simulink library "RLSUpdate_ul"  (R2018a)
settings: Solver=VariableStepAuto  StartTime=0.0  StopTime=10.0  RelTol=1e-3
undefined symbols (not defined in the file or in its folder): p
settings Model: Creator=mitch  LastModifiedBy=mitch

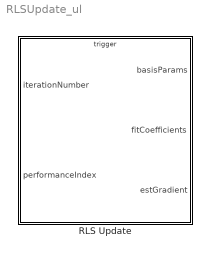
== system RLSUpdate_ul ==
  RLS Update : Subsystem  TreatAsAtomicUnit=on  mask{settlingBasisParameter=0, initializationBasisParameters=p.initializationBasisParameters*pi/180, numSettlingLaps=p.numSettlingLaps, forgettingFactor=p.forgettingFactor, normalizationFactors=p.basisParameterNormalizationFactors'*pi/180, trustRegionDimensions=p.trustRegionDimensions'*pi/180, learningGain=p.KLearningGradient, noiseAmplitude=0}
      mask prompts: settlingBasisParameter "Settling Basis Parameters"; initializationBasisParameters "Initialization Basis Parameters"; numSettlingLaps "Number of Settling Laps"; forgettingFactor "Forgetting Factor"; normalizationFactors "Basis Parameter Normalization Factors"; trustRegionDimensions "Trust Region Dimensions"; learningGain "Learning Gain"; noiseAmplitude "Noise Amplitudes"
      mask help:
      | Block implementing my RLS update
      | All vectors must be columns
      | See help for detailed description of inputs
      mask Help:
      | RLS update of the basis parameters using a quadratic regressor vector and gradient based update with a trust region.
      | let N be the number of basis parameters and M be the number of points in basis parameter design space used to initialize the algorithm
      | 
      | INPUTS :
      | Initialization basis parameters - M by N matrix where each row contains a combination of basis parameters used to initalizat the algorithm
      | Number of settling laps - scalar number of laps before initialization phase
      | Forgetting Factor - scalar forgetting factor between 0 and 1
      | Basis Parameters Normalization Factors - N by 1 matrix (vector) where each element is the relative sensitivity to that basis parameter (higher means less sensitive).  Each element can also be thought of as the characteristic change in that basis parameter necessary to produce similiar change in the overall performance.
      | Trust Region Dimensions - N by 1 matrix (vector) that limits movement between iterations
      | Learning Gain - scalar gain used to multiply the gradient before applying the trust region limits.

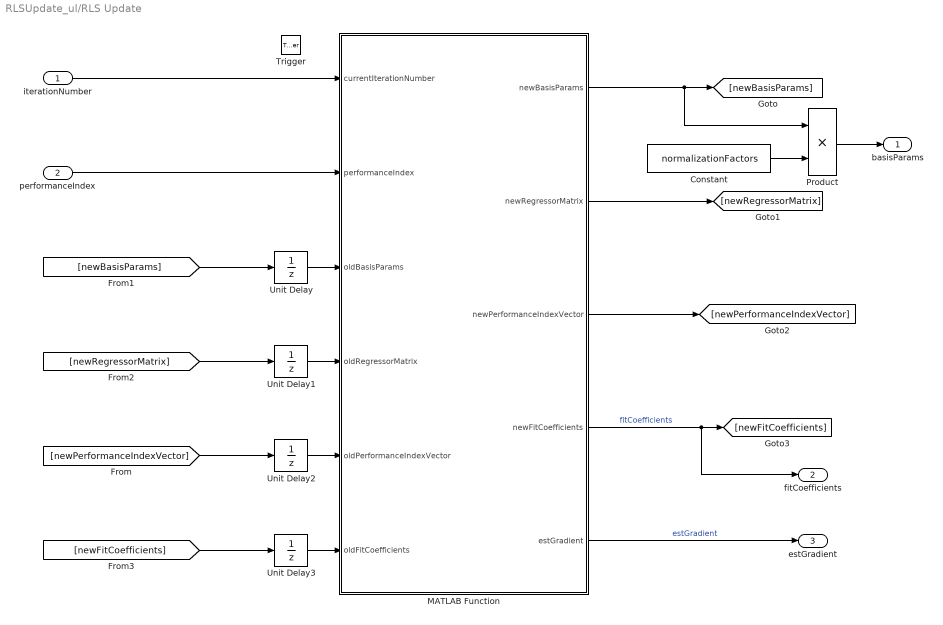
== system RLSUpdate_ul/RLS Update ==
  iterationNumber : Inport
  performanceIndex : Inport  Port=2
  Trigger : TriggerPort  VariantControl=Variant  PortDimensions=1
  Constant : Constant  Value=normalizationFactors
  MATLAB Function : MATLAB Function  TreatAsAtomicUnit=on
  Product : Product
  Unit Delay : UnitDelay  InitialCondition=settlingBasisParameter./normalizationFactors  SampleTime=-1
  Unit Delay1 : UnitDelay  InitialCondition=nan(size(p.initializationBasisParameters,1))  SampleTime=-1
  Unit Delay2 : UnitDelay  InitialCondition=nan(size(initializationBasisParameters,1),1)  SampleTime=-1
  Unit Delay3 : UnitDelay  InitialCondition=nan(size(initializationBasisParameters,1),1)  SampleTime=-1
  basisParams : Outport  InitialOutput=settlingBasisParameter
  fitCoefficients : Outport  Port=2
  estGradient : Outport  Port=3
  wires:
  MATLAB Function/5(estGradient) -> estGradient/1  "estGradient"
  performanceIndex/1 -> MATLAB Function/2(performanceIndex)
  MATLAB Function/1(newBasisParams) -> Product/1, [newBasisParams]
  Unit Delay/1 -> MATLAB Function/3(oldBasisParams)
  [newBasisParams] -> Unit Delay/1
  Unit Delay1/1 -> MATLAB Function/4(oldRegressorMatrix)
  MATLAB Function/2(newRegressorMatrix) -> [newRegressorMatrix]
  [newRegressorMatrix] -> Unit Delay1/1
  iterationNumber/1 -> MATLAB Function/1(currentIterationNumber)
  MATLAB Function/3(newPerformanceIndexVector) -> [newPerformanceIndexVector]
  [newPerformanceIndexVector] -> Unit Delay2/1
  Unit Delay2/1 -> MATLAB Function/5(oldPerformanceIndexVector)
  MATLAB Function/4(newFitCoefficients) -> fitCoefficients/1, [newFitCoefficients]  "fitCoefficients"
  Unit Delay3/1 -> MATLAB Function/6(oldFitCoefficients)
  [newFitCoefficients] -> Unit Delay3/1
  Product/1 -> basisParams/1
  Constant/1 -> Product/2

== matlab function RLSUpdate_ul/RLS Update/MATLAB Function ==
  data: currentIterationNumber input; performanceIndex input; oldBasisParams input size=size(initializationBasisParameters(1,:)'); newBasisParams output; oldRegressorMatrix input; oldPerformanceIndexVector input; oldFitCoefficients input; newRegressorMatrix output; newPerformanceIndexVector output size=[size(initializationBasisParameters,1),1]; newFitCoefficients output; initializationBasisParameters parameter; numSettlingLaps parameter; forgettingFactor parameter; normalizationFactors parameter; trustRegionDimensions parameter; learningGain parameter; estGradient output; noiseAmplitude parameter
function [newBasisParams,newRegressorMatrix,newPerformanceIndexVector,...
    newFitCoefficients,estGradient]...
    = updateBasisParameters(...
    currentIterationNumber, performanceIndex,...
    oldBasisParams, oldRegressorMatrix,oldPerformanceIndexVector,...
    oldFitCoefficients, initializationBasisParameters, numSettlingLaps,...
    forgettingFactor, normalizationFactors, trustRegionDimensions,...
    learningGain, noiseAmplitude)

% Note all vectors are columns
numInitializationLaps = size(initializationBasisParameters,1);
numBasisParams = numel(oldBasisParams);
simulationPhase =  'settling';

if currentIterationNumber>numSettlingLaps
    simulationPhase =  'initialization';
end

if currentIterationNumber>numSettlingLaps+numInitializationLaps
    simulationPhase = 'optimization';
end

switch simulationPhase
    case 'settling'
        newBasisParams      = oldBasisParams;
        newRegressorMatrix  = oldRegressorMatrix;
        newPerformanceIndexVector = nan(numInitializationLaps,1);
        newFitCoefficients        = nan(numInitializationLaps,1);
        estGradient = nan(numBasisParams,1);
        
    case 'initialization'
        initializationIndex = currentIterationNumber - numInitializationLaps;
        newBasisParams      = initializationBasisParameters(initializationIndex,:)'./normalizationFactors;
        newRegressorMatrix  = oldRegressorMatrix;
        newRegressorMatrix(initializationIndex,:) = buildRegressorVector(newBasisParams)';
        newPerformanceIndexVector = oldPerformanceIndexVector;
        if initializationIndex>1
            newPerformanceIndexVector(initializationIndex-1) = performanceIndex;
        end
        newFitCoefficients = nan(numInitializationLaps,1);
        estGradient = nan(numBasisParams,1);
        
    case 'optimization'
        if currentIterationNumber == numSettlingLaps+ numInitializationLaps + 1
            % If it's the first time through, solve least squares
            newPerformanceIndexVector = oldPerformanceIndexVector;
            newPerformanceIndexVector(end) = performanceIndex;
            R = oldRegressorMatrix;
            newRegressorMatrix  = (R'*R)\R';
            x = newPerformanceIndexVector;
            newFitCoefficients = newRegressorMatrix*x;
        else
            % Otherwise, do the RLS update
            % https://en.wikipedia.org/wiki/Recursive_least_squares_filter
            x = buildRegressorVector(oldBasisParams)';
            w = oldFitCoefficients;
            d = performanceIndex;
            P = oldRegressorMatrix;
            f = forgettingFactor;
            alpha = d - x'*w;
            g = P*x*(f+x'*P*x)^-1;
            P = (f^-1)*(P-g*x'*(f^-1)*P);
            w = w +alpha*g;
            newFitCoefficients = w;
            newRegressorMatrix = P;
        end
        
        estGradient = [...
            newFitCoefficients(2)+2*newFitCoefficients(3)*oldBasisParams(1)...
            newFitCoefficients(4)+2*newFitCoefficients(5)*oldBasisParams(2)]';
        % Normalize the gradient
        %         estGradient = estGradient/norm(estGradient);
        
        
        updateGradient = learningGain*estGradient;
        normalizedTrustRegion = (trustRegionDimensions)./normalizationFactors;
        trustRegionGain = min([1 ...
            normalizedTrustRegion(1)/abs(updateGradient(1))...
            normalizedTrustRegion(2)/abs(updateGradient(2))]);
        
        newBasisParams      = oldBasisParams+trustRegionGain*updateGradient...
            + noiseAmplitude.*(2*rand(size(oldBasisParams))-1);
        newPerformanceIndexVector = nan(numInitializationLaps,1);
        
    otherwise
        newBasisParams      = nan(numBasisParams,1);
        newRegressorMatrix  = nan(numInitializationLaps);
        newPerformanceIndexVector = nan(numInitializationLaps,1);
        newFitCoefficients     = nan(numInitializationLaps,1);
        estGradient = nan(numBasisParams,1);
end
end

function vec = buildRegressorVector(basisParams)
vec = nan(1+2*numel(basisParams),1)';
vec(1) = 1;
for ii = 2:2:1+2*numel(basisParams)
    vec(ii) = basisParams(ii/2);
    vec(ii+1) = basisParams(ii/2)^2;
end
end
